simulink model "MST_AyrikModel_2022"  (R2022b)
settings: Solver=FixedStepAuto  StartTime=0.0  StopTime=10.0  FixedStep=0.1  RelTol=1e-3
InitFcn:
  | MST_Ayrik
undefined symbols (not defined in the file): constants
settings Model: Creator=aysen

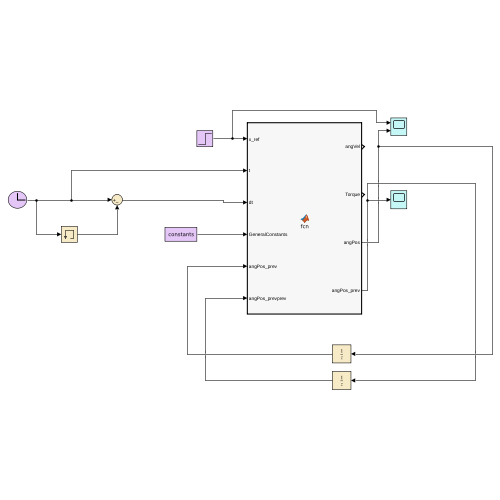
[thumbnail: Simulink's stored preview of the top-level diagram]
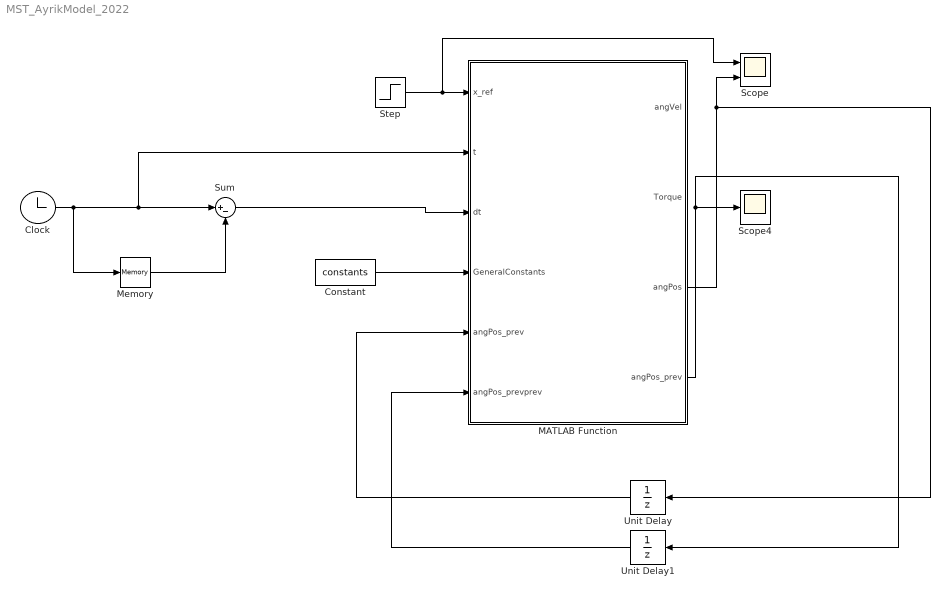
== system MST_AyrikModel_2022 ==
  Clock : Clock
  Constant : Constant  Value=constants
  MATLAB Function : MATLAB Function  TreatAsAtomicUnit=on
  Memory : Memory
  Scope : Scope  NumInputPorts=2
  Scope4 : Scope
  Step : Step  Time=0  After=10  SampleTime=0
  Sum : Sum  Inputs=|+-
  Unit Delay : UnitDelay  SampleTime=-1  HasFrameUpgradeWarning=on
  Unit Delay1 : UnitDelay  SampleTime=-1  HasFrameUpgradeWarning=on
  wires:
  Clock/1 -> Memory/1, MATLAB Function/2(t), Sum/1
  Memory/1 -> Sum/2
  Sum/1 -> MATLAB Function/3(dt)
  Constant/1 -> MATLAB Function/4(GeneralConstants)
  MATLAB Function/3(angPos) -> Unit Delay/1, Scope/2
  Unit Delay/1 -> MATLAB Function/5("angPos_prev ")
  Unit Delay1/1 -> MATLAB Function/6(angPos_prevprev)
  MATLAB Function/4(angPos_prev) -> Unit Delay1/1, Scope4/1
  Step/1 -> Scope/1, MATLAB Function/1(x_ref)

== matlab function MST_AyrikModel_2022/MATLAB Function ==
  data: angVel output; Torque output size=1; x_ref input size=1; angPos output size=1; angPos_prev output; t input size=1; dt input; GeneralConstants input; angPos_prev input size=1; angPos_prevprev input size=1
function [angVel, Torque, angPos, angPos_prev] = fcn(x_ref,t, dt, GeneralConstants, angPos_prev, angPos_prevprev)
fx_now = GeneralConstants(1,1);
fx_pre = GeneralConstants(2,1);
fx_fut = GeneralConstants(3,1);
x_0 = GeneralConstants(4,1);
x_0_dot = GeneralConstants(5, 1);
Ae = GeneralConstants(6, 1);

error = x_ref - angPos_prev;
C1 = x_ref - (((angPos_prev * fx_now) + (angPos_prevprev * fx_pre)) / fx_fut);

if (t == 0)
    angPos = x_0;       
    angVel = 0;
    Torque = 0;

elseif (t == dt)
    Torque = fx_fut * (C1 - (Ae * error));
    angPos = x_0 + x_0_dot * dt;
    angVel = x_0_dot;

else
    Torque = fx_fut * (C1 - (Ae * error));
    angPos = (angPos_prev * fx_now + angPos_prevprev * fx_pre + Torque) / fx_fut;
    angVel = (angPos - angPos_prevprev) / (2 * dt);
    Torque = Torque * 1000;
end
